simulink model "AM_DSB_SC_DEMODULATION"  (R2024a)
settings: Solver=VariableStepAuto  StartTime=0.0  StopTime=10.0  RelTol=1e-3
libraries: dspfdesign x1
settings Model: Creator=zeyad  LastModifiedBy=zeyad

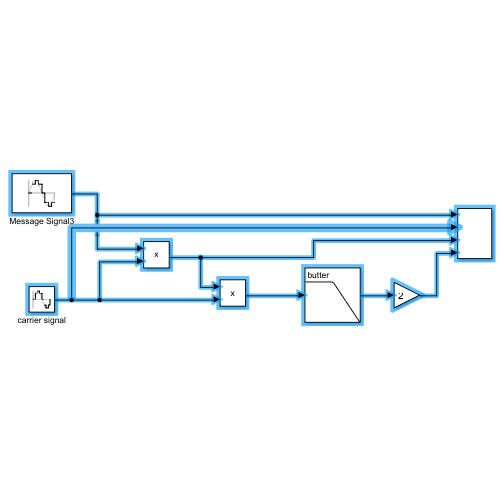
[thumbnail: Simulink's stored preview of the top-level diagram]
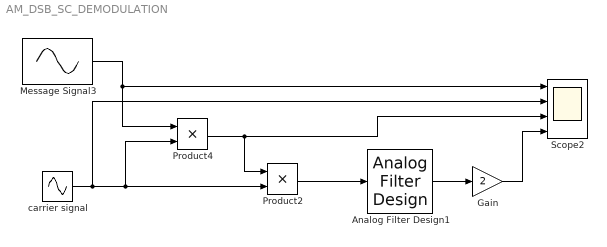
== system AM_DSB_SC_DEMODULATION ==
  Analog Filter Design1 : dspfdesign/Analog Filter Design  method=Butterworth  filttype=Lowpass  N=8  Wlo=60  Whi=80  Rp=2  Rs=40
  Gain : Gain  Gain=2
  Message Signal3 : Sin  Frequency=5  SampleTime=1/1000
  Product2 : Product
  Product4 : Product
  Scope2 : Scope  NumInputPorts=4
  carrier signal : Sin  Frequency=50  SampleTime=1/1000
  wires:
  Gain/1 -> Scope2/4
  Analog Filter Design1/1 -> Gain/1
  Message Signal3/1 -> Product4/1, Scope2/1
  Product2/1 -> Analog Filter Design1/1
  Product4/1 -> Product2/1, Scope2/3
  carrier signal/1 -> Scope2/2, Product2/2, Product4/2
